simulink model "Pendulum"  (R2014a)
settings: Solver=ode45  StartTime=0.0  StopTime=10.0  RelTol=1e-3
values from neighbouring files (symbols this model uses):
  H = place( A',C', Polos_OB )'    [script_8.m]
  k = place( A ,B , Polos_CO )    [script_8.m]
undefined symbols (not defined in the file or in its folder): A, B, C, D
settings Model: Creator=matlab  LastModifiedBy=matlab

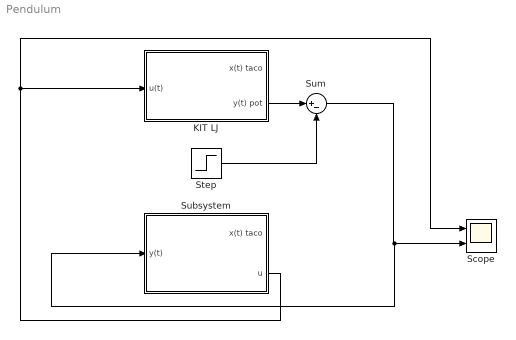
== system Pendulum ==
  KIT LJ : Subsystem
  Scope : Scope  NumInputPorts=2
      settings: YMin=-5~-5  YMax=5~5
  Step : Step  SampleTime=0
  Subsystem : Subsystem
  Sum : Sum  Inputs=|+-
  wires:
  KIT LJ/2(y(t) pot) -> Sum/1
  Sum/1 -> Subsystem/1(y(t)), Scope/2
  Step/1 -> Sum/2
  Subsystem/2(u) -> Scope/1, KIT LJ/1(u(t))

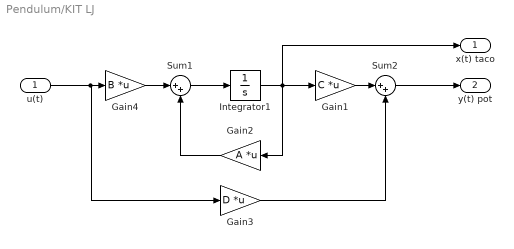
== system Pendulum/KIT LJ ==
  u(t) : Inport
  Gain1 : Gain  Gain=C  Multiplication=Matrix(K*u)
  Gain2 : Gain  Gain=A  Multiplication=Matrix(K*u)
  Gain3 : Gain  Gain=D  Multiplication=Matrix(K*u)
  Gain4 : Gain  Gain=B  Multiplication=Matrix(K*u)
  Integrator1 : Integrator
  Sum1 : Sum  Inputs=|++
  Sum2 : Sum  Inputs=|++
  x(t) taco : Outport
  y(t) pot : Outport  Port=2
  wires:
  Gain4/1 -> Sum1/1
  Integrator1/1 -> x(t) taco/1, Gain2/1, Gain1/1
  Sum1/1 -> Integrator1/1
  Gain2/1 -> Sum1/2
  Sum2/1 -> y(t) pot/1
  Gain1/1 -> Sum2/1
  Gain3/1 -> Sum2/2
  u(t)/1 -> Gain3/1, Gain4/1

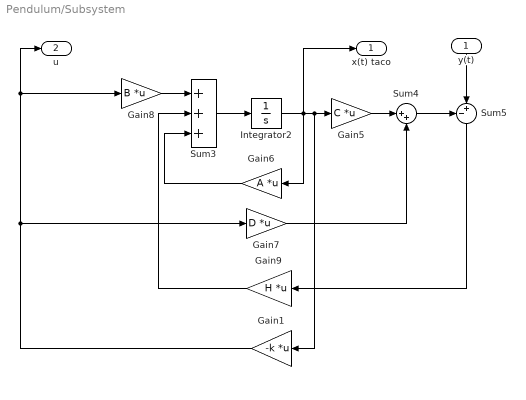
== system Pendulum/Subsystem ==
  y(t) : Inport
  Gain1 : Gain  Gain=-k  Multiplication=Matrix(K*u)
  Gain5 : Gain  Gain=C  Multiplication=Matrix(K*u)
  Gain6 : Gain  Gain=A  Multiplication=Matrix(K*u)
  Gain7 : Gain  Gain=D  Multiplication=Matrix(K*u)
  Gain8 : Gain  Gain=B  Multiplication=Matrix(K*u)
  Gain9 : Gain  Gain=H  Multiplication=Matrix(K*u)
  Integrator2 : Integrator
  Sum3 : Sum  Inputs=+++
  Sum4 : Sum  Inputs=|++
  Sum5 : Sum  Inputs=-+|
  x(t) taco : Outport
  u : Outport  Port=2
  wires:
  Gain6/1 -> Sum3/3
  Gain9/1 -> Sum3/2
  Integrator2/1 -> x(t) taco/1, Gain1/1, Gain5/1, Gain6/1
  Sum4/1 -> Sum5/1
  Sum5/1 -> Gain9/1
  Sum3/1 -> Integrator2/1
  Gain7/1 -> Sum4/2
  Gain5/1 -> Sum4/1
  Gain8/1 -> Sum3/1
  y(t)/1 -> Sum5/2
  Gain1/1 -> u/1, Gain8/1, Gain7/1
